simulink subsystem "DC_Motor"  (R2023a)
settings: Solver=VariableStepAuto  StartTime=0.0  StopTime=10.0  RelTol=1e-3
values from neighbouring files (symbols this model uses):
  J_motor = 500 * 10^-9    (= 5e-07)    [constants.m]
  km = 16 * 10^-3    (= 0.016)    [constants.m]
  kw = 1 / (20 * pi)    (= 0.0159154943092)    [constants.m]
  L = 350 * 10^-6    (= 0.00035)    [constants.m]
  R_dc = 10    [constants.m]
  vis_friction_coef_motor = 0.05    [constants.m]
settings Model: Creator=ПК  LastModifiedBy=ycheb

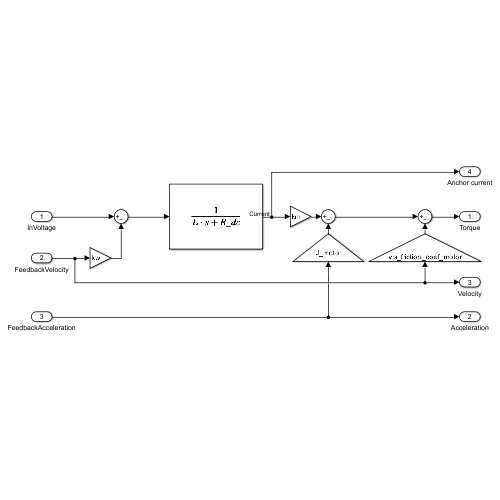
[thumbnail: Simulink's stored preview of the top-level diagram]
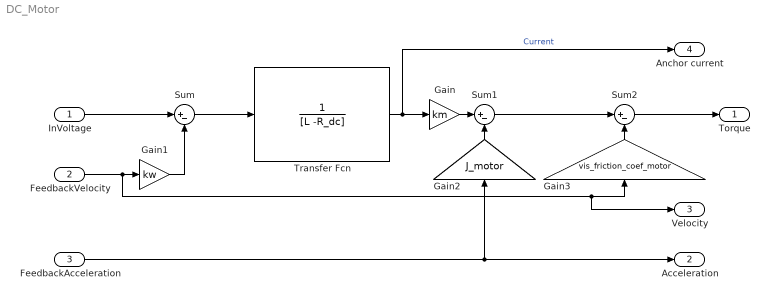
== system DC_Motor ==
  InVoltage : Inport
  FeedbackVelocity : Inport  Port=2
  FeedbackAcceleration : Inport  Port=3
  Gain : Gain  Gain=km
  Gain1 : Gain  Gain=kw
  Gain2 : Gain  Gain=J_motor
  Gain3 : Gain  Gain=vis_friction_coef_motor
  Sum : Sum  Inputs=|+-
  Sum1 : Sum  Inputs=|+-
  Sum2 : Sum  Inputs=|+-
  Transfer Fcn : TransferFcn  Denominator=[L -R_dc]
  Torque : Outport
  Acceleration : Outport  Port=2
  Velocity : Outport  Port=3
  Anchor current : Outport  Port=4
  wires:
  Sum/1 -> Transfer Fcn/1
  Transfer Fcn/1 -> Anchor current/1, Gain/1  "Current"
  Gain1/1 -> Sum/2
  FeedbackAcceleration/1 -> Gain2/1, Acceleration/1
  Gain/1 -> Sum1/1
  Gain2/1 -> Sum1/2
  Sum1/1 -> Sum2/1
  Gain3/1 -> Sum2/2
  FeedbackVelocity/1 -> Gain3/1, Velocity/1, Gain1/1
  InVoltage/1 -> Sum/1
  Sum2/1 -> Torque/1
